simulink model "PubIfDecisionTOS_MDL"  (R2020b)
settings: configuration reference "DspaceConfig" (kept outside this file)
PostLoadFcn:
  | if any(exist('dsrtsu_mdlpostloadfcn', 'file') ~= 0), dsrtsu_mdlpostloadfcn('Execute', bdroot); end
InitFcn:
  | , if any(exist('dsmpb_private', 'file') ~= 0), dsmpb_private('dsmpb_mdlclblib', 'Init', bdroot); end,
undefined symbols (not defined in the file or in its folder): C_TOS_ACCEgoRAxletoFbumplength_m, C_TOS_ACCTargetFront_Flag, C_TOS_AEBJAPedObjDxThre_Val, C_TOS_AEBJAPedObjDyThre_Val, C_TOS_AEBJATargetSize_Val, C_TOS_AEBJAVehObjDxThre_Val, C_TOS_AEBJAVehObjDyThre_Val, C_TOS_AEBJuncPedTargetSize_Val, C_TOS_AEBLatObjDxThre_Val, C_TOS_AEBLatPedDyThre_Val, C_TOS_AEBLatTargetSize_Val, C_TOS_AEBLongTargetInEgoFront_Flag, C_TOS_axAbsGround_Parameter, C_TOS_CameraConfirmedFlag, C_TOS_CNsubjWidth, C_TOS_CurrentLaneCoreMinWidth_Val, C_TOS_CutInProb_Val_Zero, C_TOS_CutOutProb_Val_Zero, C_TOS_D2R_Val, C_TOS_DefaultValueObjectToCenterLine_dy, C_TOS_EgoCarWidth_Val, C_TOS_EgoDxRefPoint_m, C_TOS_EgoRAxletoFbumplength_m, C_TOS_HalfWidthVehicle_Con, C_TOS_HWA_CurrentLaneFlag, C_TOS_HWA_LeftLaneFlag, C_TOS_HWA_MovingDir_Vaild, C_TOS_HWA_MovState_Vaild, C_TOS_HWA_RightLaneFlag, C_TOS_LaneLineCourseErrorFront, C_TOS_LaneLineCourseErrorRear, C_TOS_MotorbikeDefaultWidth_m, C_TOS_NumberOfEffectiveTargets, C_TOS_Obj_Age_Val, C_TOS_Objdx_Constraint_Val, C_TOS_ObjectDefaultWidth_m, C_TOS_ObjInCurrentLane_Val, C_TOS_ObjInCurrentLaneValid, C_TOS_ObjInLeftLaneValid, C_TOS_ObjInRightLaneValid, C_TOS_ObjNotInCurrentLane_Val, C_TOS_ObjNotREElementType, C_TOS_ObjPredictDis_dy_ConstantVal_Zeros, C_TOS_ObjToCenterLine_ConstantVal_Zeros, C_TOS_OFMObjIDInvilad_Val, C_TOS_PIL_LatDisCons_Val_zero, C_TOS_PIL_ObjectCutInFlag_b, C_TOS_PIL_ObjectCutOutFlag_b, C_TOS_PIL_ObjLaneProb_al_Val, C_TOS_PP_ObjFusType_FC_Confirm_b, C_TOS_PP_ObjFusType_FC_FR_Confirm_b, C_TOS_PP_ObjFusType_FR_Confirm_b, C_TOS_RE_80BoolDefault_Val, C_TOS_RE_80Single181Default_Val, C_TOS_RE_80Single255Default_Val, C_TOS_RE_80Uint8Default_Val, C_TOS_RE_D2R, C_TOS_RE_D_180_Val, C_TOS_RE_InvalidObjectID_Val, C_TOS_RE_InvalidTargetChainDir_Val ... (+142)
libraries: simulink x1650, TOS_LIB x361, canfdmsglib x14
(part 41 of 69)

== system PubIfDecisionTOS_MDL/TOS_20201112/TOS_2012080320/PIL_1029/ObjCutInOut_Prob/ObjectCutIn/CutInProb_Calculate/CutInProb_Calculate_/CutInProb_ScopeConstraint1/ObjectCutinMind1/CutInObjWidthConstraint ==
  note: 根据目标宽度，修正切入预测距离
  note: 目标在中心线左侧
  note: 目标在中心线右侧
  ObjectToCenterLine_dy : Inport  OutDataTypeStr=single
  Object_Width : Inport  Port=2
  Abs2 : Abs
  Add : Sum  Inputs=-+
  Add1 : Sum
  C_HalfWidthVehicle_Con : Constant  Value=C_TOS_HalfWidthVehicle_Con  OutDataTypeStr=single
      settings: AttributesFormatString=C_TOS_HalfWidthVehicle_Con = 0.5
  Compare To Constant2 : simulink/Logic and Bit Operations/Compare To Constant  relop=<=  const=P_TOS_CutinObjectToCenterLine_dy_Val  OutDataTypeStr=boolean
      settings: AttributesFormatString=P_TOS_CutinObjectToCenterLine_dy_Val = 0.1
  Constant3 : Constant  Value=C_TOS_ObjToCenterLine_ConstantVal_Zeros  OutDataTypeStr=single
      settings: AttributesFormatString=C_TOS_ObjToCenterLine_ConstantVal_Zeros = 0
  Max : MinMax  Function=max  Inputs=2  OutDataTypeStr=single
  Max1 : MinMax  Inputs=2  OutDataTypeStr=single
  Product : Product  OutDataTypeStr=single
  Relational Operator : RelationalOperator  Operator=>  OutDataTypeStr=boolean  RndMeth=Nearest
  Switch : Switch  Criteria=u2 > Threshold  OutDataTypeStr=single
  constant1 : Constant  Value=0  OutDataTypeStr=single
  constant2 : Constant  Value=0  OutDataTypeStr=single
  CutInPredictDis_dy_ObjWidthConstraint : Outport
  wires:
  Add1/1 -> Max1/2
  Product/1 -> Add/1, Add1/2
  C_HalfWidthVehicle_Con/1 -> Product/1
  Relational Operator/1 -> Switch/2
  Constant3/1 -> Relational Operator/2
  constant1/1 -> Max/1
  ObjectToCenterLine_dy/1 -> Add/2, Add1/1, Relational Operator/1
  Object_Width/1 -> Product/2
  Max/1 -> Switch/1
  constant2/1 -> Max1/1
  Max1/1 -> Switch/3
  Add/1 -> Max/2
  Switch/1 -> Abs2/1
  Abs2/1 -> Compare To Constant2/1
  Compare To Constant2/1 -> CutInPredictDis_dy_ObjWidthConstraint/1

== system PubIfDecisionTOS_MDL/TOS_20201112/TOS_2012080320/PIL_1029/ObjCutInOut_Prob/ObjectCutOut/CutOutProb_Calculate/CutOutProb_Calculate/CutOutPredictDis_dy/CutOutPredictTime/CarTruck_ToCenterLine_dy_Predict ==
  ObjectType : Inport
  PP_ObjectToCenterLine_vyc : Inport  Port=2  OutDataTypeStr=single
  Abs : Abs
  Compare To Constant : simulink/Logic and Bit Operations/Compare To Constant  relop===  const=OFM_OBJ_TYPE_E.CAR  OutDataTypeStr=boolean
      settings: AttributesFormatString=OFM_OBJ_TYPE_E.CAR = 2
  Compare To Constant1 : simulink/Logic and Bit Operations/Compare To Constant  relop===  const=OFM_OBJ_TYPE_E.TRUCK  OutDataTypeStr=boolean
      settings: AttributesFormatString=OFM_OBJ_TYPE_E.TRUCK = 3
  Compare To Constant2 : simulink/Logic and Bit Operations/Compare To Constant  relop=>  const=P_TOS_CutinObjvyThre_CarTruck_Val  OutDataTypeStr=boolean
      settings: AttributesFormatString=P_TOS_CutinObjvyThre_CarTruck_Val = 0.1
  Data Type Conversion : DataTypeConversion  OutDataTypeStr=Enum: OFM_OBJ_TYPE_E
  Logical Operator1 : Logic  AllPortsSameDT=off  OutDataTypeStr=boolean
  Logical Operator16 : Logic  Operator=OR  AllPortsSameDT=off  OutDataTypeStr=boolean
  CarTruck_ToCenterLine_dy_Predict : Outport
  wires:
  ObjectType/1 -> Data Type Conversion/1
  Logical Operator16/1 -> Logical Operator1/1
  Compare To Constant1/1 -> Logical Operator16/2
  Compare To Constant/1 -> Logical Operator16/1
  PP_ObjectToCenterLine_vyc/1 -> Abs/1
  Compare To Constant2/1 -> Logical Operator1/2
  Abs/1 -> Compare To Constant2/1
  Logical Operator1/1 -> CarTruck_ToCenterLine_dy_Predict/1
  Data Type Conversion/1 -> Compare To Constant1/1, Compare To Constant/1

== system PubIfDecisionTOS_MDL/TOS_20201112/TOS_2012080320/PIL_1029/ObjCutInOut_Prob/ObjectCutOut/CutOutProb_Calculate/CutOutProb_Calculate/CutOutPredictDis_dy/CutOutPredictTime/ObjectToCenterLine_dy_Predict ==
  note: 当前值 - 滤波后值
  note: 目标在中心线右侧
  note: 目标在中心线左侧
  note: 根据 ObjectToCenterLine_dy 定义CutOut预测时间
  ObjectToCenterLine_dy_Filt : Inport  OutDataTypeStr=single
  ObjectToCenterLine_dy : Inport  Port=2  OutDataTypeStr=single
  Add : Sum  Inputs=-+  OutDataTypeStr=single
  Compare To Constant : simulink/Logic and Bit Operations/Compare To Constant  relop=<  const=C_TOS_ObjToCenterLine_ConstantVal_Zeros  OutDataTypeStr=boolean
      settings: AttributesFormatString=C_TOS_ObjToCenterLine_ConstantVal_Zeros = 0
  Compare To Constant1 : simulink/Logic and Bit Operations/Compare To Constant  relop=<  const=P_TOS_CutOut_ObjectToCenterLine_Rightdy_Con  OutDataTypeStr=boolean
      settings: AttributesFormatString=P_TOS_CutOut_ObjectToCenterLine_Rightdy_Con = -0.1
  Compare To Constant2 : simulink/Logic and Bit Operations/Compare To Constant  relop=>=  const=P_TOS_CutOut_ObjectToCenterLine_Leftdy_Con  OutDataTypeStr=boolean
      settings: AttributesFormatString=P_TOS_CutOut_ObjectToCenterLine_Leftdy_Con = 0.1
  Compare To Constant3 : simulink/Logic and Bit Operations/Compare To Constant  relop=>=  const=C_TOS_ObjToCenterLine_ConstantVal_Zeros  OutDataTypeStr=boolean
      settings: AttributesFormatString=C_TOS_ObjToCenterLine_ConstantVal_Zeros = 0
  K_CutInMaxPredictTime_Val : Constant  Value=P_TOS_CutOutMaxPredictTime_Val  OutDataTypeStr=single
      settings: AttributesFormatString=P_TOS_CutOutMaxPredictTime_Val = 1.0
  K_CutInMinPredictTime_Val : Constant  Value=P_TOS_CutOutMinPredictTime_Val  OutDataTypeStr=single
      settings: AttributesFormatString=P_TOS_CutOutMinPredictTime_Val = 0
  Logical Operator : Logic  AllPortsSameDT=off  OutDataTypeStr=boolean
  Logical Operator1 : Logic  Operator=OR  AllPortsSameDT=off  OutDataTypeStr=boolean
  Logical Operator2 : Logic  AllPortsSameDT=off  OutDataTypeStr=boolean
  Switch : Switch  Criteria=u2 > Threshold  OutDataTypeStr=single
  CutOutPredictTime : Outport
  wires:
  Add/1 -> Compare To Constant2/1, Compare To Constant1/1
  K_CutInMinPredictTime_Val/1 -> Switch/3
  K_CutInMaxPredictTime_Val/1 -> Switch/1
  Compare To Constant1/1 -> Logical Operator2/2
  ObjectToCenterLine_dy_Filt/1 -> Add/1
  Compare To Constant/1 -> Logical Operator2/1
  Logical Operator/1 -> Logical Operator1/2
  [ObjectToCenterLine_dy] -> Compare To Constant3/1
  [ObjectToCenterLine_dy] -> Compare To Constant/1
  Compare To Constant2/1 -> Logical Operator/1
  Logical Operator2/1 -> Logical Operator1/1
  Logical Operator1/1 -> Switch/2
  Switch/1 -> CutOutPredictTime/1  "CutOutPredictTime"
  Compare To Constant3/1 -> Logical Operator/2
  ObjectToCenterLine_dy/1 -> [ObjectToCenterLine_dy], Add/2

== system PubIfDecisionTOS_MDL/TOS_20201112/TOS_2012080320/PIL_1029/ObjCutInOut_Prob/ObjectCutOut/CutOutProb_Calculate/CutOutProb_Calculate/CutOutProb/CutOutObjWidthConstraint/ObjectWidth_Check ==
  ObjectType : Inport
  Object_Width : Inport  Port=2
  Compare To Constant : simulink/Logic and Bit Operations/Compare To Constant  relop===  const=OFM_OBJ_TYPE_E.CAR  OutDataTypeStr=boolean
      settings: AttributesFormatString=OFM_OBJ_TYPE_E.CAR = 2
  Compare To Constant1 : simulink/Logic and Bit Operations/Compare To Constant  relop===  const=OFM_OBJ_TYPE_E.TRUCK  OutDataTypeStr=boolean
      settings: AttributesFormatString=OFM_OBJ_TYPE_E.TRUCK = 3
  Compare To Constant2 : simulink/Logic and Bit Operations/Compare To Constant  relop===  const=OFM_OBJ_TYPE_E.MOTORBIKE  OutDataTypeStr=boolean
      settings: AttributesFormatString=OFM_OBJ_TYPE_E.MOTORBIKE = 4
  Constant : Constant  Value=C_TOS_MotorbikeDefaultWidth_m  OutDataTypeStr=single
      settings: AttributesFormatString=C_TOS_MotorbikeDefaultWidth_m = 1
  Constant1 : Constant  Value=C_TOS_ObjectDefaultWidth_m  OutDataTypeStr=single
      settings: AttributesFormatString=C_TOS_ObjectDefaultWidth_m = 0.5
  Data Type Conversion : DataTypeConversion  OutDataTypeStr=Enum: OFM_OBJ_TYPE_E
  Logical Operator16 : Logic  Operator=OR  AllPortsSameDT=off  OutDataTypeStr=boolean
  Saturation : Saturate  UpperLimit=2.4  LowerLimit=1.6  OutDataTypeStr=single
  Switch : Switch  Criteria=u2 > Threshold
  Switch1 : Switch  Criteria=u2 > Threshold
  ObjectWidth : Outport
  wires:
  Constant1/1 -> Switch1/3
  Constant/1 -> Switch1/1
  Compare To Constant2/1 -> Switch1/2
  Switch1/1 -> Switch/3
  Saturation/1 -> Switch/1
  Switch/1 -> ObjectWidth/1
  Object_Width/1 -> Saturation/1
  ObjectType/1 -> Data Type Conversion/1
  Logical Operator16/1 -> Switch/2
  Compare To Constant1/1 -> Logical Operator16/2
  Data Type Conversion/1 -> Compare To Constant1/1, Compare To Constant2/1, Compare To Constant/1
  Compare To Constant/1 -> Logical Operator16/1

== system PubIfDecisionTOS_MDL/TOS_20201112/TOS_2012080320/PIL_1029/ObjCutInOut_Prob/ObjectCutOut/CutOutProb_Calculate/CutOutProb_Calculate/CutOutProb_ScopeConstraint/ObjectCutoutMind/CutOutObjCutinMov ==
  note: 根据目标宽度，修正切入预测距离
  PP_ObjectToCenterLine_vyc : Inport
  ObjectToCenterLine_dy : Inport  Port=2  OutDataTypeStr=single
  Compare To Constant1 : simulink/Logic and Bit Operations/Compare To Constant  relop=>  const=C_TOS_ObjToCenterLine_ConstantVal_Zeros  OutDataTypeStr=boolean
      settings: AttributesFormatString=C_TOS_ObjToCenterLine_ConstantVal_Zeros = 0
  Constant : Constant  Value=P_TOS_CutoutObjvyThre_Val  OutDataTypeStr=single
      settings: AttributesFormatString=P_TOS_CutoutObjvyThre_Val = 0.1
  Constant1 : Constant  Value=P_TOS_CutoutObjvyThre_Val  OutDataTypeStr=single
      settings: AttributesFormatString=P_TOS_CutoutObjvyThre_Val = 0.1
  Gain : Gain  Gain=-1
  Relational Operator1 : RelationalOperator  Operator=<=  OutDataTypeStr=boolean  RndMeth=Nearest
  Relational Operator2 : RelationalOperator  OutDataTypeStr=boolean  RndMeth=Nearest
  Switch : Switch  Criteria=u2 ~= 0
  CutOutObjCutinMovflg : Outport
  wires:
  Switch/1 -> CutOutObjCutinMovflg/1
  ObjectToCenterLine_dy/1 -> Compare To Constant1/1
  Compare To Constant1/1 -> Switch/2
  Constant/1 -> Gain/1
  PP_ObjectToCenterLine_vyc/1 -> Relational Operator2/1, Relational Operator1/1
  Gain/1 -> Relational Operator1/2
  Relational Operator1/1 -> Switch/1
  Constant1/1 -> Relational Operator2/2
  Relational Operator2/1 -> Switch/3

== system PubIfDecisionTOS_MDL/TOS_20201112/TOS_2012080320/PIL_1029/ObjCutInOut_Prob/ObjectCutOut/CutOutProb_Calculate/CutOutProb_Calculate/CutOutProb_ScopeConstraint/ObjectCutoutMind/CutOutObjWidthConstraint ==
  note: 调节目标释放时机
  note: <1.5m时，不计算cut out概率值
  note: 目标在中心线左侧
  note: 目标在中心线右侧
  PP_ObjectToCenterLine_dy : Inport  OutDataTypeStr=single
  Object_Width : Inport  Port=2
  ObjectType : Inport  Port=3
  Abs2 : Abs  OutDataTypeStr=single
  Add : Sum  Inputs=-+
  Add1 : Sum
  C_HalfWidthVehicle_Con : Constant  Value=C_TOS_HalfWidthVehicle_Con  OutDataTypeStr=single
      settings: AttributesFormatString=C_TOS_HalfWidthVehicle_Con = 0.5
  Constant1 : Constant  Value=P_TOS_CutoutBoundaryToCenterLine_Val  OutDataTypeStr=single
      settings: AttributesFormatString=P_TOS_CutoutBoundaryToCenterLine_Val = 1.5
  Constant3 : Constant  Value=C_TOS_ObjToCenterLine_ConstantVal_Zeros  OutDataTypeStr=single
      settings: AttributesFormatString=C_TOS_ObjToCenterLine_ConstantVal_Zeros = 0
  Max : MinMax  Function=max  Inputs=2  OutDataTypeStr=single
  Max1 : MinMax  Inputs=2  OutDataTypeStr=single
  ObjectWidth_Check : Subsystem
  Product : Product  OutDataTypeStr=single
  Relational Operator : RelationalOperator  Operator=>  OutDataTypeStr=boolean  RndMeth=Nearest
  Relational Operator2 : RelationalOperator  Operator=<=  OutDataTypeStr=boolean  RndMeth=Nearest
  Switch : Switch  Criteria=u2 ~= 0  OutDataTypeStr=single
  constant1 : Constant  Value=0  OutDataTypeStr=single
  constant2 : Constant  Value=0  OutDataTypeStr=single
  CutOutPredictDis_dy_ObjWidthConstraint : Outport
  wires:
  ObjectType/1 -> ObjectWidth_Check/1(ObjectType)
  Object_Width/1 -> ObjectWidth_Check/2(Object_Width)
  Add1/1 -> Max1/2
  Product/1 -> Add/1, Add1/2
  C_HalfWidthVehicle_Con/1 -> Product/1
  Relational Operator/1 -> Switch/2
  Constant3/1 -> Relational Operator/2
  constant1/1 -> Max/1
  PP_ObjectToCenterLine_dy/1 -> Add/2, Add1/1, Relational Operator/1
  ObjectWidth_Check/1(ObjectWidth) -> Product/2
  Max/1 -> Switch/1
  constant2/1 -> Max1/1
  Max1/1 -> Switch/3
  Add/1 -> Max/2
  Switch/1 -> Abs2/1
  Abs2/1 -> Relational Operator2/1
  Constant1/1 -> Relational Operator2/2
  Relational Operator2/1 -> CutOutPredictDis_dy_ObjWidthConstraint/1

== system PubIfDecisionTOS_MDL/TOS_20201112/TOS_2012080320/PP1128/AAT-AdditionalAttributes/RoadEdge/RE_2020_12_07/RoadEdge_V2/RoadEdgeElementFinalJudge/EgoLeft_RoadEdgeElementsFinalJudge/Dy_Filter ==
  Object_Dy : Inport  Partition=on  PartitionDimension=1  PartitionWidth=1  PartitionOffset=0
  Object_Dy_K1 : Inport  Port=2  Partition=on  PartitionDimension=1  PartitionWidth=1  PartitionOffset=0
  RE_EdgeElementID_K1 : Inport  Port=3  Partition=on  PartitionDimension=1  PartitionWidth=1  PartitionOffset=0
  Object_ID : Inport  Port=4  Partition=on  PartitionDimension=1  PartitionWidth=1  PartitionOffset=0
  Compare To Constant : simulink/Logic and Bit Operations/Compare To Constant  relop===  const=C_TOS_RE_InvalidObjectID_Val  OutDataTypeStr=boolean
      settings: AttributesFormatString=%<const> = 0
  For Each : ForEach  DisableCoverage=on
  If : If  NumInputs=2  IfExpression=u1|u2
  If Action Subsystem : Subsystem  TreatAsAtomicUnit=on
  Merge : Merge
  Relational Operator : RelationalOperator  Operator=~=  OutDataTypeStr=boolean  RndMeth=Simplest
  Subsystem : Subsystem
  Object_DyFilter : Outport  ConcatenationDimension=1
  wires:
  Object_ID/1 -> Relational Operator/1, Compare To Constant/1
  Compare To Constant/1 -> If/1
  Object_Dy/1 -> [Object_Dy], Subsystem/1(Object_Dy)
  Object_Dy_K1/1 -> Subsystem/2(Object_Dy_K1)
  Subsystem/1(Object_DyFilter) -> Merge/2
  If/2 -> Subsystem/Action
  If/1 -> If Action Subsystem/Action
  If Action Subsystem/1(Object_DyFilter) -> Merge/1
  Merge/1 -> Object_DyFilter/1
  [Object_Dy] -> If Action Subsystem/1(Object_Dy)
  RE_EdgeElementID_K1/1 -> Relational Operator/2
  Relational Operator/1 -> If/2

== system PubIfDecisionTOS_MDL/TOS_20201112/TOS_2012080320/PP1128/AAT-AdditionalAttributes/RoadEdge/RE_2020_12_07/RoadEdge_V2/RoadEdgeElementFinalJudge/EgoLeft_RoadEdgeElementsFinalJudge/For Each Subsystem ==
  RE_EdgeElementFlag : Inport  Partition=on  PartitionDimension=1  PartitionWidth=1  PartitionOffset=0
  Compare To Constant : simulink/Logic and Bit Operations/Compare To Constant  relop===  const=4  OutDataTypeStr=boolean
  For Each : ForEach  DisableCoverage=on
  Sum of Elements : Sum  Inputs=+
  Tapped Delay : simulink/Discrete/Tapped Delay  vinit=0.0  samptime=-1  NumDelays=3  DelayOrder=Oldest  includeCurrent=on
  RE_4StepEdgeElementFlag : Outport  ConcatenationDimension=1
  wires:
  Sum of Elements/1 -> Compare To Constant/1
  Compare To Constant/1 -> RE_4StepEdgeElementFlag/1
  Tapped Delay/1 -> Sum of Elements/1
  RE_EdgeElementFlag/1 -> Tapped Delay/1  "EdgeElementFlag"

== system PubIfDecisionTOS_MDL/TOS_20201112/TOS_2012080320/PP1128/AAT-AdditionalAttributes/RoadEdge/RE_2020_12_07/RoadEdge_V2/RoadEdgeElementFinalJudge/EgoLeft_RoadEdgeElementsFinalJudge/RoadEdgeElementFinalJudge/RoadEdgeElementInJudge.RoadEdgeElementTheta1Cal.TargetDisJudge ==
  note: 当相邻两个元素，或相隔两个元素之间DxDy间距很小时，Dx<5m,8m.Dy<0.5m,0.8m.阈值的Offset经过查表得到
  Target4_Dy : Inport  OutDataTypeStr=single  PortDimensions=1
  Target3_Dy : Inport  Port=2  OutDataTypeStr=single  PortDimensions=1
  Target1_Dy : Inport  Port=3  OutDataTypeStr=single  PortDimensions=1
  Target4_Dx : Inport  Port=4  OutDataTypeStr=single  PortDimensions=1
  Target3_Dx : Inport  Port=5  OutDataTypeStr=single  PortDimensions=1
  Target1_Dx : Inport  Port=6  OutDataTypeStr=single  PortDimensions=1
  f : TriggerPort  TriggerType=function-call  VariantControl=(inherit)
      settings: CopyFcn=Stateflow.SLINSF.SimulinkMan.removeBlockPreDeleteFcn  PreDeleteFcn=Stateflow.SLINSF.SimulinkMan.unsafePredeleteFcn
  1-D Lookup Table : Lookup_n-D  NumberOfTableDimensions=1  BreakpointsForDimension1=[0,0.05,0.1,0.15,0.2,0.4,0.6,0.8,1,2,3,4,5,5.1,5.2]  Table=[23,23,22,21,20,15,10,9,6,5,4,3,0,0,0]  InternalRulePriority=Speed  RndMeth=Simplest  InputSameDT=on
  1-D Lookup Table1 : Lookup_n-D  NumberOfTableDimensions=1  BreakpointsForDimension1=[0,0.1,0.2,0.3,0.4,0.8,1.2,1.6,2,4,6,8,10,10.1,10.2]  Table=[23,23,22,21,20,15,10,9,6,5,4,3,0,0,0]  InternalRulePriority=Speed  RndMeth=Simplest  InputSameDT=on
  Abs{,1..3} (4 alike) : Abs
  Add{,1..3} (4 alike) : Sum  Inputs=+-
  Compare To Constant : simulink/Logic and Bit Operations/Compare To Constant  relop=<=  const=P_TOS_RE_NebrNearTargetDxThre_Val  OutDataTypeStr=boolean
      settings: AttributesFormatString=%<const> = 5
  Compare To Constant1 : simulink/Logic and Bit Operations/Compare To Constant  relop=<=  const=P_TOS_RE_ApartNearTargetDxThre_Val  OutDataTypeStr=boolean
      settings: AttributesFormatString=%<const> = 8
  Compare To Constant2 : simulink/Logic and Bit Operations/Compare To Constant  relop=<  const=P_TOS_RE_ApartNearTargetDyThre_Val  OutDataTypeStr=boolean
      settings: AttributesFormatString=%<const> = 0.5
  Compare To Constant3 : simulink/Logic and Bit Operations/Compare To Constant  relop=<  const=P_TOS_RE_NebrNearTargetDyThre_Val  OutDataTypeStr=boolean
      settings: AttributesFormatString=%<const> = 0.5
  Logical Operator : Logic  Operator=OR  AllPortsSameDT=off  OutDataTypeStr=boolean
  Logical Operator1 : Logic  AllPortsSameDT=off  OutDataTypeStr=boolean
  Logical Operator2 : Logic  Operator=OR  AllPortsSameDT=off  OutDataTypeStr=boolean
  Max : MinMax  Function=max  Inputs=2
  RE_TooNear2Target_Flag : Outport
  P_RE_NearTargetThetaOffset : Outport  Port=2
  wires:
  Target3_Dx/1 -> Add2/2, Add1/1
  Target1_Dx/1 -> Add1/2
  Target4_Dx/1 -> Add2/1
  Add2/1 -> Abs/1
  Add1/1 -> Abs1/1
  Abs/1 -> 1-D Lookup Table/1, Compare To Constant/1
  Abs1/1 -> 1-D Lookup Table1/1, Compare To Constant1/1
  Compare To Constant/1 -> Logical Operator/1
  Compare To Constant1/1 -> Logical Operator/2
  Logical Operator/1 -> Logical Operator1/2
  1-D Lookup Table/1 -> Max/1
  1-D Lookup Table1/1 -> Max/2
  Max/1 -> P_RE_NearTargetThetaOffset/1
  Add/1 -> Abs2/1
  Abs2/1 -> Compare To Constant2/1
  Compare To Constant2/1 -> Logical Operator2/2
  Target1_Dy/1 -> Add/2
  Target3_Dy/1 -> Add3/2, Add/1
  Logical Operator1/1 -> RE_TooNear2Target_Flag/1
  Abs3/1 -> Compare To Constant3/1
  Add3/1 -> Abs3/1
  Target4_Dy/1 -> Add3/1
  Compare To Constant3/1 -> Logical Operator2/1
  Logical Operator2/1 -> Logical Operator1/1

== system PubIfDecisionTOS_MDL/TOS_20201112/TOS_2012080320/PP1128/AAT-AdditionalAttributes/RoadEdge/RE_2020_12_07/RoadEdge_V2/RoadEdgeElementFinalJudge/EgoLeft_RoadEdgeElementsFinalJudge/RoadEdgeElementFinalJudge/RoadEdgeElementInJudge.RoadEdgeElementTheta1Cal.Theta_Cal ==
  note: Theta=atan[(Dx_2-Dx_1)/(Dy_2-Dy_1)]*180/pi
      | atan输出正负锐角，负角转换为其补角（钝角）
      | Theta取值范围[0 180]
  note: 一阶滞后滤波
  Target3_Dx : Inport  OutDataTypeStr=single  PortDimensions=1
  Target1_Dx : Inport  Port=2  OutDataTypeStr=single  PortDimensions=1
  Target3_Dy : Inport  Port=3  OutDataTypeStr=single  PortDimensions=1
  Target1_Dy : Inport  Port=4  OutDataTypeStr=single  PortDimensions=1
  ObjectsSortIndex : Inport  Port=5
  ObjectsSortIndex_K1 : Inport  Port=6
  RE_13TargetTheta_K1 : Inport  Port=7
  f : TriggerPort  TriggerType=function-call  VariantControl=Variant
      settings: CopyFcn=Stateflow.SLINSF.SimulinkMan.removeBlockPreDeleteFcn  PreDeleteFcn=Stateflow.SLINSF.SimulinkMan.unsafePredeleteFcn
  Abs : Abs
  Add : Sum  Inputs=+-
  Add1 : Sum  Inputs=+-
  Add2 : Sum
  Add3 : Sum  Inputs=+-
  Add4 : Sum
  Compare To Constant : simulink/Logic and Bit Operations/Compare To Constant  relop=<  const=0.001  OutDataTypeStr=boolean
  Compare To Zero : simulink/Logic and Bit Operations/Compare To Zero  relop=>=  OutDataTypeStr=boolean
  Constant : Constant  Value=C_TOS_RE_D2R
      settings: AttributesFormatString=%<Value> = 180/pi
  Constant1 : Constant  Value=C_TOS_RE_D_180_Val
      settings: AttributesFormatString=%<Value> = 180
  Constant2 : Constant  Value=0.001  OutDataTypeStr=single
  Divide : Product  Inputs=*/
  Gain : Gain  Gain=0.5
  Product : Product
  Relational Operator : RelationalOperator  Operator===  OutDataTypeStr=boolean  RndMeth=Simplest
  Saturation1 : Saturate  UpperLimit=1.6331e+16  LowerLimit=-1.6331e+16
  Switch : Switch  Criteria=u2 ~= 0
  Switch1 : Switch  Criteria=u2 ~= 0
  Switch2 : Switch  Criteria=u2 ~= 0
  Trigonometric Function : Trigonometry  Operator=atan
  StillTarget13_Theta : Outport  OutDataTypeStr=single  PortDimensions=1
  wires:
  Target3_Dy/1 -> Add/1
  Target1_Dy/1 -> Add/2
  Target3_Dx/1 -> Add1/1
  Target1_Dx/1 -> Add1/2
  Add1/1 -> Divide/1
  Divide/1 -> Saturation1/1
  Trigonometric Function/1 -> Product/1
  Constant/1 -> Product/2
  Product/1 -> Switch/1, Add2/1, Compare To Zero/1
  Compare To Zero/1 -> Switch/2
  Constant1/1 -> Add2/2
  Add2/1 -> Switch/3
  Constant2/1 -> Switch1/1
  Abs/1 -> Compare To Constant/1
  Compare To Constant/1 -> Switch1/2
  Add/1 -> Switch1/3, Abs/1
  Switch1/1 -> Divide/2
  Saturation1/1 -> Trigonometric Function/1
  RE_13TargetTheta_K1/1 -> Add4/2, Add3/2
  Add4/1 -> Switch2/1
  Gain/1 -> Add4/1
  Add3/1 -> Gain/1
  Switch/1 -> Switch2/3, Add3/1  "StillTarget12_0_Theta"
  Switch2/1 -> StillTarget13_Theta/1
  ObjectsSortIndex_K1/1 -> Relational Operator/2
  ObjectsSortIndex/1 -> Relational Operator/1
  Relational Operator/1 -> Switch2/2

== system PubIfDecisionTOS_MDL/TOS_20201112/TOS_2012080320/PP1128/AAT-AdditionalAttributes/RoadEdge/RE_2020_12_07/RoadEdge_V2/RoadEdgeElementFinalJudge/EgoRight_RoadEdgeElementsFinalJudge/Dy_Filter ==
  Object_Dy : Inport  Partition=on  PartitionDimension=1  PartitionWidth=1  PartitionOffset=0
  Object_Dy_K1 : Inport  Port=2  Partition=on  PartitionDimension=1  PartitionWidth=1  PartitionOffset=0
  RE_EdgeElementID_K1 : Inport  Port=3  Partition=on  PartitionDimension=1  PartitionWidth=1  PartitionOffset=0
  Object_ID : Inport  Port=4  Partition=on  PartitionDimension=1  PartitionWidth=1  PartitionOffset=0
  Compare To Constant : simulink/Logic and Bit Operations/Compare To Constant  relop===  const=C_TOS_RE_InvalidObjectID_Val  OutDataTypeStr=boolean
      settings: AttributesFormatString=%<const> = 0
  For Each : ForEach  DisableCoverage=on
  If : If  NumInputs=2  IfExpression=u1|u2
  If Action Subsystem : Subsystem  TreatAsAtomicUnit=on
  Merge : Merge
  Relational Operator : RelationalOperator  Operator=~=  OutDataTypeStr=boolean  RndMeth=Simplest
  Subsystem : Subsystem
  Object_DyFilter : Outport  ConcatenationDimension=1
  wires:
  Object_ID/1 -> Relational Operator/1, Compare To Constant/1
  Compare To Constant/1 -> If/1
  Object_Dy/1 -> [Object_Dy], Subsystem/1(Object_Dy)
  Object_Dy_K1/1 -> Subsystem/2(Object_Dy_K1)
  Subsystem/1(Object_DyFilter) -> Merge/2
  If/2 -> Subsystem/Action
  If/1 -> If Action Subsystem/Action
  If Action Subsystem/1(Object_DyFilter) -> Merge/1
  Merge/1 -> Object_DyFilter/1
  [Object_Dy] -> If Action Subsystem/1(Object_Dy)
  RE_EdgeElementID_K1/1 -> Relational Operator/2
  Relational Operator/1 -> If/2

== system PubIfDecisionTOS_MDL/TOS_20201112/TOS_2012080320/PP1128/AAT-AdditionalAttributes/RoadEdge/RE_2020_12_07/RoadEdge_V2/RoadEdgeElementFinalJudge/EgoRight_RoadEdgeElementsFinalJudge/For Each Subsystem ==
  RE_EdgeElementFlag : Inport  Partition=on  PartitionDimension=1  PartitionWidth=1  PartitionOffset=0
  Compare To Constant : simulink/Logic and Bit Operations/Compare To Constant  relop===  const=4  OutDataTypeStr=boolean
  For Each : ForEach  DisableCoverage=on
  Sum of Elements : Sum  Inputs=+
  Tapped Delay : simulink/Discrete/Tapped Delay  vinit=0.0  samptime=-1  NumDelays=3  DelayOrder=Oldest  includeCurrent=on
  RE_4StepEdgeElementFlag : Outport  ConcatenationDimension=1
  wires:
  RE_EdgeElementFlag/1 -> Tapped Delay/1  "EdgeElementFlag"
  Tapped Delay/1 -> Sum of Elements/1
  Compare To Constant/1 -> RE_4StepEdgeElementFlag/1
  Sum of Elements/1 -> Compare To Constant/1

== system PubIfDecisionTOS_MDL/TOS_20201112/TOS_2012080320/PP1128/AAT-AdditionalAttributes/RoadEdge/RE_2020_12_07/RoadEdge_V2/RoadEdgeElementFinalJudge/EgoRight_RoadEdgeElementsFinalJudge/RoadEdgeElementFinalJudge/RoadEdgeElementInJudge.RoadEdgeElementTheta1Cal.TargetDisJudge ==
  note: 当相邻两个元素，或相隔两个元素之间DxDy间距很小时，Dx<5m,8m.Dy<0.5m,0.8m.阈值的Offset经过查表得到
  Target4_Dy : Inport  OutDataTypeStr=single  PortDimensions=1
  Target3_Dy : Inport  Port=2  OutDataTypeStr=single  PortDimensions=1
  Target1_Dy : Inport  Port=3  OutDataTypeStr=single  PortDimensions=1
  Target4_Dx : Inport  Port=4  OutDataTypeStr=single  PortDimensions=1
  Target3_Dx : Inport  Port=5  OutDataTypeStr=single  PortDimensions=1
  Target1_Dx : Inport  Port=6  OutDataTypeStr=single  PortDimensions=1
  f : TriggerPort  TriggerType=function-call  VariantControl=(inherit)
      settings: CopyFcn=Stateflow.SLINSF.SimulinkMan.removeBlockPreDeleteFcn  PreDeleteFcn=Stateflow.SLINSF.SimulinkMan.unsafePredeleteFcn
  1-D Lookup Table : Lookup_n-D  NumberOfTableDimensions=1  BreakpointsForDimension1=[0,0.05,0.1,0.15,0.2,0.4,0.6,0.8,1,2,3,4,5,5.1,5.2]  Table=[23,23,22,21,20,15,10,9,6,5,4,3,0,0,0]  InternalRulePriority=Speed  RndMeth=Simplest  InputSameDT=on
  1-D Lookup Table1 : Lookup_n-D  NumberOfTableDimensions=1  BreakpointsForDimension1=[0,0.1,0.2,0.3,0.4,0.8,1.2,1.6,2,4,6,8,10,10.1,10.2]  Table=[23,23,22,21,20,15,10,9,6,5,4,3,0,0,0]  InternalRulePriority=Speed  RndMeth=Simplest  InputSameDT=on
  Abs{,1..3} (4 alike) : Abs
  Add{,1..3} (4 alike) : Sum  Inputs=+-
  Compare To Constant : simulink/Logic and Bit Operations/Compare To Constant  relop=<=  const=P_TOS_RE_NebrNearTargetDxThre_Val  OutDataTypeStr=boolean
      settings: AttributesFormatString=%<const> = 5
  Compare To Constant1 : simulink/Logic and Bit Operations/Compare To Constant  relop=<=  const=P_TOS_RE_ApartNearTargetDxThre_Val  OutDataTypeStr=boolean
      settings: AttributesFormatString=%<const> = 8
  Compare To Constant2 : simulink/Logic and Bit Operations/Compare To Constant  relop=<  const=P_TOS_RE_ApartNearTargetDyThre_Val  OutDataTypeStr=boolean
      settings: AttributesFormatString=%<const> = 0.5
  Compare To Constant3 : simulink/Logic and Bit Operations/Compare To Constant  relop=<  const=P_TOS_RE_NebrNearTargetDyThre_Val  OutDataTypeStr=boolean
      settings: AttributesFormatString=%<const> = 0.5
  Logical Operator : Logic  Operator=OR  AllPortsSameDT=off  OutDataTypeStr=boolean
  Logical Operator1 : Logic  AllPortsSameDT=off  OutDataTypeStr=boolean
  Logical Operator2 : Logic  Operator=OR  AllPortsSameDT=off  OutDataTypeStr=boolean
  Max : MinMax  Function=max  Inputs=2
  RE_TooNear2Target_Flag : Outport
  P_RE_NearTargetThetaOffset : Outport  Port=2
  wires:
  Target3_Dx/1 -> Add2/2, Add1/1
  Target1_Dx/1 -> Add1/2
  Target4_Dx/1 -> Add2/1
  Add2/1 -> Abs/1
  Add1/1 -> Abs1/1
  Abs/1 -> 1-D Lookup Table/1, Compare To Constant/1
  Abs1/1 -> 1-D Lookup Table1/1, Compare To Constant1/1
  Compare To Constant/1 -> Logical Operator/1
  Compare To Constant1/1 -> Logical Operator/2
  Logical Operator/1 -> Logical Operator1/2
  1-D Lookup Table/1 -> Max/1
  1-D Lookup Table1/1 -> Max/2
  Max/1 -> P_RE_NearTargetThetaOffset/1
  Add/1 -> Abs2/1
  Abs2/1 -> Compare To Constant2/1
  Compare To Constant2/1 -> Logical Operator2/2
  Target1_Dy/1 -> Add/2
  Target3_Dy/1 -> Add3/2, Add/1
  Logical Operator1/1 -> RE_TooNear2Target_Flag/1
  Abs3/1 -> Compare To Constant3/1
  Add3/1 -> Abs3/1
  Target4_Dy/1 -> Add3/1
  Compare To Constant3/1 -> Logical Operator2/1
  Logical Operator2/1 -> Logical Operator1/1

== system PubIfDecisionTOS_MDL/TOS_20201112/TOS_2012080320/PP1128/AAT-AdditionalAttributes/RoadEdge/RE_2020_12_07/RoadEdge_V2/RoadEdgeElementFinalJudge/EgoRight_RoadEdgeElementsFinalJudge/RoadEdgeElementFinalJudge/RoadEdgeElementInJudge.RoadEdgeElementTheta1Cal.Theta_Cal ==
  note: Theta=atan[(Dx_2-Dx_1)/(Dy_2-Dy_1)]*180/pi
      | atan输出正负锐角，负角转换为其补角（钝角）
      | Theta取值范围[0 180]
  note: 一阶滞后滤波
  Target3_Dx : Inport  OutDataTypeStr=single  PortDimensions=1
  Target1_Dx : Inport  Port=2  OutDataTypeStr=single  PortDimensions=1
  Target3_Dy : Inport  Port=3  OutDataTypeStr=single  PortDimensions=1
  Target1_Dy : Inport  Port=4  OutDataTypeStr=single  PortDimensions=1
  ObjectsSortIndex : Inport  Port=5
  ObjectsSortIndex_K1 : Inport  Port=6
  RE_13TargetTheta_K1 : Inport  Port=7
  f : TriggerPort  TriggerType=function-call  VariantControl=Variant
      settings: CopyFcn=Stateflow.SLINSF.SimulinkMan.removeBlockPreDeleteFcn  PreDeleteFcn=Stateflow.SLINSF.SimulinkMan.unsafePredeleteFcn
  Abs : Abs
  Add : Sum  Inputs=+-
  Add1 : Sum  Inputs=+-
  Add2 : Sum
  Add3 : Sum  Inputs=+-
  Add4 : Sum
  Compare To Constant : simulink/Logic and Bit Operations/Compare To Constant  relop=<  const=0.001  OutDataTypeStr=boolean
  Compare To Zero : simulink/Logic and Bit Operations/Compare To Zero  relop=>=  OutDataTypeStr=boolean
  Constant : Constant  Value=C_TOS_RE_D2R
      settings: AttributesFormatString=%<Value> = 180/pi
  Constant1 : Constant  Value=C_TOS_RE_D_180_Val
      settings: AttributesFormatString=%<Value> = 180
  Constant2 : Constant  Value=0.001  OutDataTypeStr=single
  Divide : Product  Inputs=*/
  Gain : Gain  Gain=0.5
  Product : Product
  Relational Operator : RelationalOperator  Operator===  OutDataTypeStr=boolean  RndMeth=Simplest
  Saturation1 : Saturate  UpperLimit=1.6331e+16  LowerLimit=-1.6331e+16
  Switch : Switch  Criteria=u2 ~= 0
  Switch1 : Switch  Criteria=u2 ~= 0
  Switch2 : Switch  Criteria=u2 ~= 0
  Trigonometric Function : Trigonometry  Operator=atan
  StillTarget13_Theta : Outport  OutDataTypeStr=single  PortDimensions=1
  wires:
  Target3_Dy/1 -> Add/1
  Target1_Dy/1 -> Add/2
  Target3_Dx/1 -> Add1/1
  Target1_Dx/1 -> Add1/2
  Add1/1 -> Divide/1
  Divide/1 -> Saturation1/1
  Trigonometric Function/1 -> Product/1
  Constant/1 -> Product/2
  Product/1 -> Switch/1, Add2/1, Compare To Zero/1
  Compare To Zero/1 -> Switch/2
  Constant1/1 -> Add2/2
  Add2/1 -> Switch/3
  Constant2/1 -> Switch1/1
  Abs/1 -> Compare To Constant/1
  Compare To Constant/1 -> Switch1/2
  Add/1 -> Switch1/3, Abs/1
  Switch1/1 -> Divide/2
  Saturation1/1 -> Trigonometric Function/1
  RE_13TargetTheta_K1/1 -> Add4/2, Add3/2
  Add4/1 -> Switch2/1
  Gain/1 -> Add4/1
  Add3/1 -> Gain/1
  Switch/1 -> Switch2/3, Add3/1  "StillTarget12_0_Theta"
  Switch2/1 -> StillTarget13_Theta/1
  ObjectsSortIndex_K1/1 -> Relational Operator/2
  ObjectsSortIndex/1 -> Relational Operator/1
  Relational Operator/1 -> Switch2/2

== system PubIfDecisionTOS_MDL/TOS_20201112/TOS_2012080320/PP1128/AAT-AdditionalAttributes/RoadEdge/RE_2020_12_07/RoadEdge_V2/SelectStationaryObjects/SelectStationaryObject/RE_StationaryObjectsSortCond ==
  note: 筛选符合如下条件目标：
      | [1]FR_Other
      | [2] fus.object.stand_b = True;
      | [3]-100m<dx<200m;
      | [4]-20m<dy<20m;
      | [5]dxv 的方差小于 12.5 ；
      | [6]dyv 的方差小于 12.5;
  Object_FusType : Inport
  Object_MovingState : Inport  Port=2
  Object_Dx : Inport  Port=3
  Object_Dy : Inport  Port=4
  Object_DxStd : Inport  Port=5
  Object_DyStd : Inport  Port=6
  Object_ExistProb : Inport  Port=7
  Object_ExistProb_K1 : Inport  Port=8
  Action Port : ActionPort  ActionPortLabel=else
  Logical Operator : Logic  Inputs=5  AllPortsSameDT=off  OutDataTypeStr=boolean
  RE_Object_DxDy : Subsystem
  RE_Object_DxDyStd : Subsystem
  RE_Object_FusType : Subsystem
  RE_Object_MovingState : Subsystem
  Subsystem : Subsystem
  RE_StationaryObjectFlag : Outport
  wires:
  RE_Object_MovingState/1(RE_Object_Stationary) -> Logical Operator/2
  RE_Object_FusType/1(RE_Object_FR_Other) -> Logical Operator/1
  RE_Object_DxDy/1(RE_Object_DxDy) -> Logical Operator/3
  Logical Operator/1 -> RE_StationaryObjectFlag/1
  RE_Object_DxDyStd/1(RE_Object_DxDyStd) -> Logical Operator/4
  Object_FusType/1 -> RE_Object_FusType/1(Object_FusType)
  Object_MovingState/1 -> RE_Object_MovingState/1(Object_MovingState)
  Object_Dx/1 -> RE_Object_DxDy/1(Object_Dx)
  Object_Dy/1 -> RE_Object_DxDy/2(Object_Dy)
  Object_DxStd/1 -> RE_Object_DxDyStd/1(Object_DxStd)
  Object_DyStd/1 -> RE_Object_DxDyStd/2(Object_DyStd)
  Object_ExistProb/1 -> Subsystem/1(Object_ExistProb)
  Subsystem/1(RE_Object_ExistProb) -> Logical Operator/5
  Object_ExistProb_K1/1 -> Subsystem/2(Object_ExistProb_K1)

== system PubIfDecisionTOS_MDL/TOS_20201112/TOS_2012080320/PP1128/AAT-AdditionalAttributes/RoadEdge/RE_2020_12_07/RoadEdge_V2/SelectStationaryObjects/SelectStationaryObject/RE_StationaryObjectsSortDefault ==
  Action Port : ActionPort  ActionPortLabel=if(u1)
  Constant : Constant  Value=0  OutDataTypeStr=boolean
  RE_StationaryObjectFlag : Outport
  wires:
  Constant/1 -> RE_StationaryObjectFlag/1

== system PubIfDecisionTOS_MDL/TOS_20201112/TOS_2012080320/PP1128/AAT-AdditionalAttributes/RoadEdge/RE_2020_12_07/RoadEdge_V2/TargetChain/EgoLeftTargetChainDirection/Dy_Filter ==
  Object_Dy : Inport  Partition=on  PartitionDimension=1  PartitionWidth=1  PartitionOffset=0
  Object_Dy_K1 : Inport  Port=2  Partition=on  PartitionDimension=1  PartitionWidth=1  PartitionOffset=0
  Object_ID : Inport  Port=3  Partition=on  PartitionDimension=1  PartitionWidth=1  PartitionOffset=0
  RE_EdgeElementID_K1 : Inport  Port=4  Partition=on  PartitionDimension=1  PartitionWidth=1  PartitionOffset=0
  Compare To Constant : simulink/Logic and Bit Operations/Compare To Constant  relop===  const=C_TOS_RE_InvalidObjectID_Val  OutDataTypeStr=boolean
      settings: AttributesFormatString=%<const> = 0
  For Each : ForEach  DisableCoverage=on
  If : If  NumInputs=2  IfExpression=u1|u2
  If Action Subsystem : Subsystem  TreatAsAtomicUnit=on
  Merge : Merge
  Relational Operator : RelationalOperator  Operator=~=  OutDataTypeStr=boolean  RndMeth=Simplest
  Subsystem : Subsystem
  Object_DyFilter : Outport  ConcatenationDimension=1
  wires:
  Object_ID/1 -> Relational Operator/1, Compare To Constant/1
  Compare To Constant/1 -> If/1
  Object_Dy/1 -> [Object_Dy], Subsystem/1(Object_Dy)
  Object_Dy_K1/1 -> Subsystem/2(Object_Dy_K1)
  Subsystem/1(Object_DyFilter) -> Merge/2
  If/2 -> Subsystem/Action
  If/1 -> If Action Subsystem/Action
  If Action Subsystem/1(Object_DyFilter) -> Merge/1
  Merge/1 -> Object_DyFilter/1
  [Object_Dy] -> If Action Subsystem/1(Object_Dy)
  RE_EdgeElementID_K1/1 -> Relational Operator/2
  Relational Operator/1 -> If/2

== system PubIfDecisionTOS_MDL/TOS_20201112/TOS_2012080320/PP1128/AAT-AdditionalAttributes/RoadEdge/RE_2020_12_07/RoadEdge_V2/TargetChain/EgoLeftTargetChainDirection/Theta_Calculation/Theta_Cal ==
  note: 一阶滞后滤波
  note: Theta=atan[(Dx_2-Dx_1)/(Dy_2-Dy_1)]*180/pi
      | atan输出正负锐角，负角转换为其补角（钝角）
      | Theta取值范围[0 180]
  ObjectsSortIndex : Inport
  ObjectsSortIndex_K1 : Inport  Port=2
  StillTarget2_Dx : Inport  Port=3  OutDataTypeStr=single  PortDimensions=1
  StillTarget1_Dx : Inport  Port=4  OutDataTypeStr=single  PortDimensions=1
  StillTarget2_Dy : Inport  Port=5  OutDataTypeStr=single  PortDimensions=1
  StillTarget1_Dy : Inport  Port=6  OutDataTypeStr=single  PortDimensions=1
  RE_2TargetTheta_K1 : Inport  Port=7
  f : TriggerPort  TriggerType=function-call  VariantControl=Variant
      settings: CopyFcn=Stateflow.SLINSF.SimulinkMan.removeBlockPreDeleteFcn  PreDeleteFcn=Stateflow.SLINSF.SimulinkMan.unsafePredeleteFcn
  Abs : Abs
  Add : Sum  Inputs=+-
  Add1 : Sum  Inputs=+-
  Add2 : Sum
  Add3 : Sum  Inputs=+-
  Add4 : Sum
  Compare To Constant : simulink/Logic and Bit Operations/Compare To Constant  relop=<  const=0.001  OutDataTypeStr=boolean
  Compare To Zero : simulink/Logic and Bit Operations/Compare To Zero  relop=>=  OutDataTypeStr=boolean
  Constant : Constant  Value=C_TOS_RE_D2R
      settings: AttributesFormatString=%<Value> = 180/pi
  Constant1 : Constant  Value=C_TOS_RE_D_180_Val
      settings: AttributesFormatString=%<Value> = 180
  Constant2 : Constant  Value=0.001  OutDataTypeStr=single
  Divide : Product  Inputs=*/
  Gain : Gain  Gain=0.5
  Product : Product
  Relational Operator : RelationalOperator  Operator===  OutDataTypeStr=boolean  RndMeth=Simplest
  Saturation1 : Saturate  UpperLimit=1.6331e+16  LowerLimit=-1.6331e+16
  Switch : Switch  Criteria=u2 ~= 0
  Switch1 : Switch  Criteria=u2 ~= 0
  Switch2 : Switch  Criteria=u2 ~= 0
  Trigonometric Function : Trigonometry  Operator=atan
  StillTarget12_0_Theta : Outport  OutDataTypeStr=single  PortDimensions=1
  wires:
  StillTarget2_Dy/1 -> Add/1
  StillTarget1_Dy/1 -> Add/2
  StillTarget2_Dx/1 -> Add1/1
  StillTarget1_Dx/1 -> Add1/2
  Add/1 -> Switch1/3, Abs/1
  Add1/1 -> Divide/1
  Switch1/1 -> Divide/2
  Divide/1 -> Saturation1/1
  Trigonometric Function/1 -> Product/1
  Constant/1 -> Product/2
  Product/1 -> Switch/1, Add2/1, Compare To Zero/1
  Compare To Zero/1 -> Switch/2
  Constant1/1 -> Add2/2
  Add2/1 -> Switch/3
  Switch/1 -> Switch2/3, Add3/1  "StillTarget12_0_Theta"
  Saturation1/1 -> Trigonometric Function/1
  Abs/1 -> Compare To Constant/1
  Compare To Constant/1 -> Switch1/2
  Constant2/1 -> Switch1/1
  ObjectsSortIndex/1 -> Relational Operator/1
  Relational Operator/1 -> Switch2/2
  Switch2/1 -> StillTarget12_0_Theta/1
  ObjectsSortIndex_K1/1 -> Relational Operator/2
  RE_2TargetTheta_K1/1 -> Add4/2, Add3/2
  Add3/1 -> Gain/1
  Gain/1 -> Add4/1
  Add4/1 -> Switch2/1

== system PubIfDecisionTOS_MDL/TOS_20201112/TOS_2012080320/PP1128/AAT-AdditionalAttributes/RoadEdge/RE_2020_12_07/RoadEdge_V2/TargetChain/EgoRightTargetChainDirection/Dy_Filter ==
  Object_Dy : Inport  Partition=on  PartitionDimension=1  PartitionWidth=1  PartitionOffset=0
  Object_Dy_K1 : Inport  Port=2  Partition=on  PartitionDimension=1  PartitionWidth=1  PartitionOffset=0
  Object_ID : Inport  Port=3  Partition=on  PartitionDimension=1  PartitionWidth=1  PartitionOffset=0
  RE_EdgeElementID_K1 : Inport  Port=4  Partition=on  PartitionDimension=1  PartitionWidth=1  PartitionOffset=0
  Compare To Constant : simulink/Logic and Bit Operations/Compare To Constant  relop===  const=C_TOS_RE_InvalidObjectID_Val  OutDataTypeStr=boolean
      settings: AttributesFormatString=%<const> = 0
  For Each : ForEach  DisableCoverage=on
  If : If  NumInputs=2  IfExpression=u1|u2
  If Action Subsystem : Subsystem  TreatAsAtomicUnit=on
  Merge : Merge
  Relational Operator : RelationalOperator  Operator=~=  OutDataTypeStr=boolean  RndMeth=Simplest
  Subsystem : Subsystem
  Object_DyFilter : Outport  ConcatenationDimension=1
  wires:
  Object_ID/1 -> Relational Operator/1, Compare To Constant/1
  Compare To Constant/1 -> If/1
  Object_Dy/1 -> [Object_Dy], Subsystem/1(Object_Dy)
  Object_Dy_K1/1 -> Subsystem/2(Object_Dy_K1)
  Subsystem/1(Object_DyFilter) -> Merge/2
  If/2 -> Subsystem/Action
  If/1 -> If Action Subsystem/Action
  If Action Subsystem/1(Object_DyFilter) -> Merge/1
  Merge/1 -> Object_DyFilter/1
  [Object_Dy] -> If Action Subsystem/1(Object_Dy)
  RE_EdgeElementID_K1/1 -> Relational Operator/2
  Relational Operator/1 -> If/2

== system PubIfDecisionTOS_MDL/TOS_20201112/TOS_2012080320/PP1128/AAT-AdditionalAttributes/RoadEdge/RE_2020_12_07/RoadEdge_V2/TargetChain/EgoRightTargetChainDirection/Theta_Calculation/Theta_Cal ==
  note: 一阶滞后滤波
  note: Theta=atan[(Dx_2-Dx_1)/(Dy_2-Dy_1)]*180/pi
      | atan输出正负锐角，负角转换为其补角（钝角）
      | Theta取值范围[0 180]
  ObjectsSortIndex : Inport
  ObjectsSortIndex_K1 : Inport  Port=2
  StillTarget2_Dx : Inport  Port=3  OutDataTypeStr=single  PortDimensions=1
  StillTarget1_Dx : Inport  Port=4  OutDataTypeStr=single  PortDimensions=1
  StillTarget2_Dy : Inport  Port=5  OutDataTypeStr=single  PortDimensions=1
  StillTarget1_Dy : Inport  Port=6  OutDataTypeStr=single  PortDimensions=1
  RE_2TargetTheta_K1 : Inport  Port=7
  f : TriggerPort  TriggerType=function-call  VariantControl=Variant
      settings: CopyFcn=Stateflow.SLINSF.SimulinkMan.removeBlockPreDeleteFcn  PreDeleteFcn=Stateflow.SLINSF.SimulinkMan.unsafePredeleteFcn
  Abs : Abs
  Add : Sum  Inputs=+-
  Add1 : Sum  Inputs=+-
  Add2 : Sum
  Add3 : Sum  Inputs=+-
  Add4 : Sum
  Compare To Constant : simulink/Logic and Bit Operations/Compare To Constant  relop=<  const=0.001  OutDataTypeStr=boolean
  Compare To Zero : simulink/Logic and Bit Operations/Compare To Zero  relop=>=  OutDataTypeStr=boolean
  Constant : Constant  Value=C_TOS_RE_D2R
      settings: AttributesFormatString=%<Value> = 180/pi
  Constant1 : Constant  Value=C_TOS_RE_D_180_Val
      settings: AttributesFormatString=%<Value> = 180
  Constant2 : Constant  Value=0.001  OutDataTypeStr=single
  Divide : Product  Inputs=*/
  Gain : Gain  Gain=0.5
  Product : Product
  Relational Operator : RelationalOperator  Operator===  OutDataTypeStr=boolean  RndMeth=Simplest
  Saturation1 : Saturate  UpperLimit=1.6331e+16  LowerLimit=-1.6331e+16
  Switch : Switch  Criteria=u2 ~= 0
  Switch1 : Switch  Criteria=u2 ~= 0
  Switch2 : Switch  Criteria=u2 ~= 0
  Trigonometric Function : Trigonometry  Operator=atan
  StillTarget12_0_Theta : Outport  OutDataTypeStr=single  PortDimensions=1
  wires:
  StillTarget2_Dy/1 -> Add/1
  StillTarget1_Dy/1 -> Add/2
  StillTarget2_Dx/1 -> Add1/1
  StillTarget1_Dx/1 -> Add1/2
  Add/1 -> Switch1/3, Abs/1
  Add1/1 -> Divide/1
  Switch1/1 -> Divide/2
  Divide/1 -> Saturation1/1
  Trigonometric Function/1 -> Product/1
  Constant/1 -> Product/2
  Product/1 -> Switch/1, Add2/1, Compare To Zero/1
  Compare To Zero/1 -> Switch/2
  Constant1/1 -> Add2/2
  Add2/1 -> Switch/3
  Switch/1 -> Switch2/3, Add3/1  "StillTarget12_0_Theta"
  Saturation1/1 -> Trigonometric Function/1
  Abs/1 -> Compare To Constant/1
  Compare To Constant/1 -> Switch1/2
  Constant2/1 -> Switch1/1
  ObjectsSortIndex/1 -> Relational Operator/1
  Relational Operator/1 -> Switch2/2
  Switch2/1 -> StillTarget12_0_Theta/1
  ObjectsSortIndex_K1/1 -> Relational Operator/2
  RE_2TargetTheta_K1/1 -> Add4/2, Add3/2
  Add3/1 -> Gain/1
  Gain/1 -> Add4/1
  Add4/1 -> Switch2/1
